simulink library "libreria_comunicaciones_servidor1"  (R2018a)
settings: Solver=VariableStepAuto  StartTime=0.0  StopTime=10.0  RelTol=1e-3
settings Model: Creator=ana-n  LastModifiedBy=ana-n
settings CodeAppCC: StateflowObjectComments=on

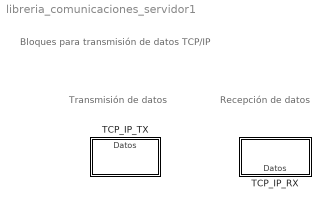
== system libreria_comunicaciones_servidor1 ==
  note: Bloques para transmisión de datos TCP/IP
  note: Recepción de datos
  note: Transmisión de datos
  TCP_IP_RX : Subsystem
      mask Display: disp('TCP_IP_RX')
  TCP_IP_TX : Subsystem
      mask Display: disp('TCP_IP_TX');

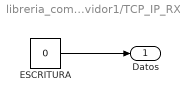
== system libreria_comunicaciones_servidor1/TCP_IP_RX ==
  ESCRITURA : Constant  Value=0
  Datos : Outport
  wires:
  ESCRITURA/1 -> Datos/1

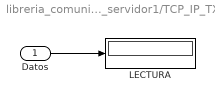
== system libreria_comunicaciones_servidor1/TCP_IP_TX ==
  Datos : Inport
  LECTURA : Display
  wires:
  Datos/1 -> LECTURA/1
